simulink model "Encoder_reader_simulink"  (R2025a)
settings: Solver=FixedStepAuto  StartTime=0.0  StopTime=inf  FixedStep=0.01  RelTol=1e-3  EnableMultiTasking=on
libraries: stm32g4xxblockslib x3, stm32f4xxblockslib x1
settings Model: STM32="{\"EncoderBlockForG4\":[{\"ID\":\"untitled:1\"},{\"ID\":\"Lab3_Encoder:1\"},{\"ID\":\"Encoder_reader_simulink:25\"},{\"ID\":\"Encoder_reader_simulink:37\"},{\"ID\":\"Encoder_reader_simulink:81\"}],\"DigitalPortRead\":{\"ID\":\"Encoder_reader_simulink:61\"}}"  Creator=User  LastModifiedBy=jua
settings OptimizationCC: DefaultParameterBehavior=Inlined  EnhancedBackFolding=on  PassReuseOutputArgsAs=Individual arguments  ZeroExternalMemoryAtStartup=off  ZeroInternalMemoryAtStartup=off  MaxStackSize=512  OptimizeBlockOrder=speed  DifferentSizesBufferReuse=on  OptimizationCustomize=off  EfficientTunableParamExpr=on
settings DebuggingCC: ParameterTunabilityLossMsg=error
settings HardwareCC: ProdBitPerPointer=32.0  ProdBitPerSizeT=32.0  ProdBitPerPtrDiffT=32.0  ProdLargestAtomicInteger=Long  ProdLargestAtomicFloat=Double  ProdWordSize=32.0  ProdLongLongMode=on  ProdHWDeviceType=ARM Compatible->ARM Cortex-M
settings SFSimCC: MATLABDynamicMemAlloc=off
settings RTWCC: SystemTargetFile=ert.tlc  HardwareBoard=STM32G4xx Based  TemplateMakefile=ert_default_tmf  Toolchain=GNU Tools for ARM Embedded Processors  Description=Embedded Coder
settings CodeAppCC: ForceParamTrailComments=on  IgnoreCustomStorageClasses=off  OperatorAnnotations=on  SimulinkDataObjDesc=on  SFDataObjDesc=on  InsertBlockDesc=on
settings ERTTargetCC: ExtModeTransport=3.0  ExtModeStaticAllocSize=2048.0  TargetLangStandard=C99 (ISO)  CodeReplacementLibrary=ARM Cortex-M  SupportContinuousTime=on

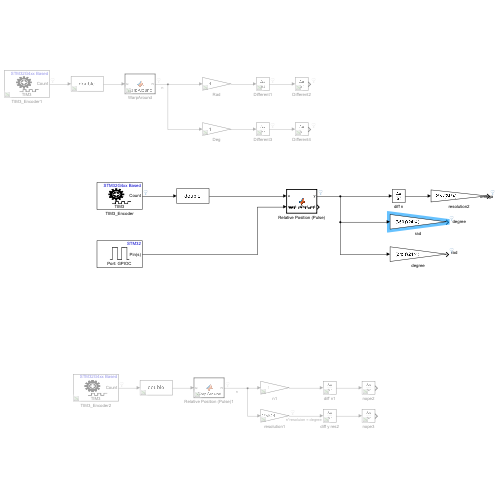
[thumbnail: Simulink's stored preview of the top-level diagram]
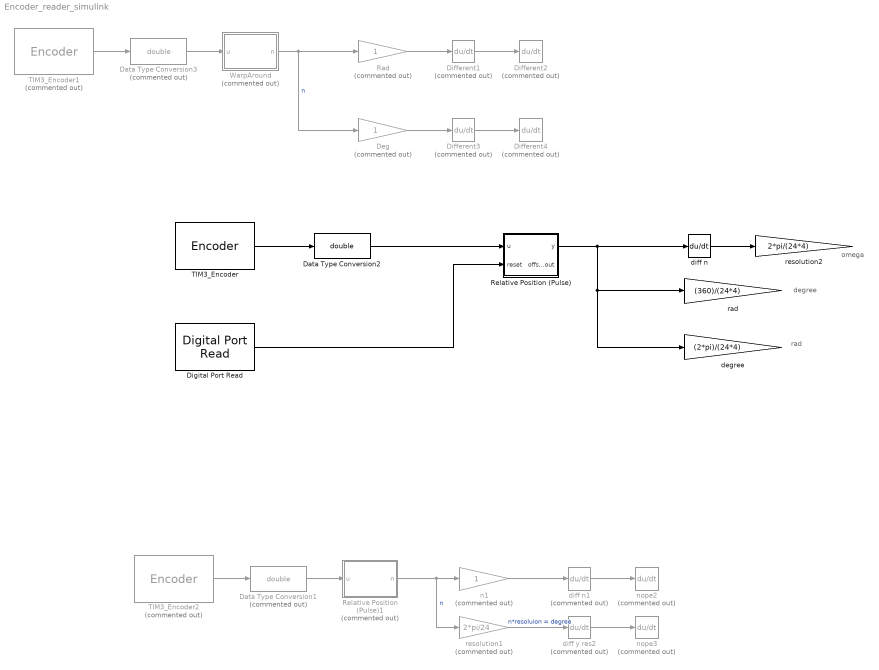
== system Encoder_reader_simulink ==
  note: degree
  note: rad
  note: omega
  Data Type Conversion1 : DataTypeConversion  Commented=on  OutDataTypeStr=double  SaturateOnIntegerOverflow=off  RndMeth=Floor
  Data Type Conversion2 : DataTypeConversion  OutDataTypeStr=double  SaturateOnIntegerOverflow=off  RndMeth=Floor
  Data Type Conversion3 : DataTypeConversion  Commented=on  OutDataTypeStr=double  SaturateOnIntegerOverflow=off  RndMeth=Floor
  Deg : Gain  Commented=on
  Different{1..4} (4 alike) : Derivative  Commented=on
  Digital Port Read : stm32f4xxblockslib/Digital Port Read  PortName=GPIOC  PinNumber=13  ReadOperation=on  IOAsArray=on  SampleTime=-1  EnableSimPort=off  hoistedMaskSrc=ECSoC/ECSimCodegen/Digital Port Read
      settings: LibrarySourceBlock=stm32g4xxblockslib/Digital Port Read
  Rad : Gain  Commented=on
  Relative Position (Pulse) : MATLAB Function  TreatAsAtomicUnit=on
  Relative Position (Pulse)1 : MATLAB Function  Commented=on  TreatAsAtomicUnit=on
  TIM3_Encoder : stm32g4xxblockslib/Encoder  TimerModule=TIM3  EnableResetInput=off  OutputCountAfterFirstIndex=off  OutputValidIndex=off  OutputDirection=off  OutputStatus=off  SampleTime=-1
  TIM3_Encoder1 : stm32g4xxblockslib/Encoder  Commented=on  TimerModule=TIM3  EnableResetInput=off  OutputCountAfterFirstIndex=off  OutputValidIndex=off  OutputDirection=off  OutputStatus=off  SampleTime=-1
  TIM3_Encoder2 : stm32g4xxblockslib/Encoder  Commented=on  TimerModule=TIM3  EnableResetInput=off  OutputCountAfterFirstIndex=off  OutputValidIndex=off  OutputDirection=off  OutputStatus=off  SampleTime=-1
  WarpAround : MATLAB Function  Commented=on  TreatAsAtomicUnit=on
  degree : Gain  Gain=(2*pi)/(24*4)
  diff n : Derivative
  diff n1 : Derivative  Commented=on
  diff y res2 : Derivative  Commented=on
  n1 : Gain  Commented=on
  nope2 : Derivative  Commented=on
  nope3 : Derivative  Commented=on
  rad : Gain  Gain=(360)/(24*4)
  resolution1 : Gain  Commented=on  Gain=2*pi/24
  resolution2 : Gain  Gain=2*pi/(24*4)
  wires:
  Relative Position (Pulse)/1(y) -> degree/1, rad/1, diff n/1
  diff n1/1 -> nope2/1
  resolution1/1 -> diff y res2/1  "n*resoluion = degree"
  TIM3_Encoder2/1 -> Data Type Conversion1/1
  Relative Position (Pulse)1/1(n) -> resolution1/1, n1/1  "n"
  n1/1 -> diff n1/1
  Data Type Conversion1/1 -> Relative Position (Pulse)1/1(u)
  diff y res2/1 -> nope3/1
  diff n/1 -> resolution2/1
  TIM3_Encoder/1 -> Data Type Conversion2/1
  Data Type Conversion2/1 -> Relative Position (Pulse)/1(u)
  Digital Port Read/1 -> Relative Position (Pulse)/2(reset)
  Different1/1 -> Different2/1
  Different3/1 -> Different4/1
  Rad/1 -> Different1/1
  Deg/1 -> Different3/1
  WarpAround/1(n) -> Deg/1, Rad/1  "n"
  TIM3_Encoder1/1 -> Data Type Conversion3/1
  Data Type Conversion3/1 -> WarpAround/1(u)

== matlab function Encoder_reader_simulink/Relative Position (Pulse) ==
  data: u input; y output; reset input; offset_out output
function [y,offset_out] = WarpAround(u, reset)

MAX_VALUE = 300;
RANGE_SIZE = MAX_VALUE + 1;
HALF_RANGE = RANGE_SIZE / 2;

persistent last_u round offset isHomed

if isempty(round)
    round = 0;
    last_u = u;
    offset = 0;
    isHomed = false;
end

delta = double(u) - double(last_u);

if delta < -HALF_RANGE
    round = round + 1;
elseif delta > HALF_RANGE
    round = round - 1;
end

continuous_pos = round * RANGE_SIZE + double(u);
last_u = u;

if reset == 1
    offset = continuous_pos;
    isHomed = true;
end

y = continuous_pos - offset;
offset_out = offset;
end

== matlab function Encoder_reader_simulink/Relative Position (Pulse)1 ==
  data: u input; n output
function n = WarpAround(u)
    
    MAX_VALUE = 300;
    RANGE_SIZE = MAX_VALUE + 1;
    HALF_RANGE = RANGE_SIZE / 2;
    

    persistent round;
    persistent last_u;
    

    if isempty(round)
        round = 0;
        last_u = u;
    end

    delta = double(u) - double(last_u);
    
    if delta < -HALF_RANGE
        round = round + 1;
    elseif delta > HALF_RANGE
        round = round - 1;
    end

    n = round * RANGE_SIZE + u;
    
    last_u = u;
    
end

== matlab function Encoder_reader_simulink/WarpAround ==
  data: u input; n output
function n = WarpAround(u)
    n=u;
end
